simulink model "pendulum"  (Simulink 8.3)
settings: Solver=ode4  StartTime=0.0  StopTime=Tmax  FixedStep=0.01  RelTol=1e-3
values from neighbouring files (symbols this model uses):
  A = [0 0 0 1.0 0 0.16983 0 0 0 0 0 ... (first row only)    [f16_init.m]    (also in pendulum_control_lmi.m = [0         0    1.0000         0; 0         0         0    1; pendulum_init.m = [0 1 0 0; pendulum_init.mat = [0 0 0 0 1 -10.95 0 24.92 0 -2.75 0 28.58 ... (16 elements, ; safety_controller_dynamics.m = [0 1 0 0)
  B = [0 0; 0 0; 0 0; 0 0; 0 0; 0 0; 0 0; 0 0; b71 0; 0 b82; 0 b92]    [f16_init.m]    (also in pendulum_control_lmi.m = [0;0;1.9400;-4.4400]; pendulum_init.m = [0 ; 1.94 ; 0 ; -4.44 ]; pendulum_init.mat = [0 1.94 0 -4.44]; pendulum_nonlinear_init.m = [0; b2; 0; -b4])
  K = K_lmi    [pendulum_init.m]    (also in pendulum_nonlinear_init.m = [7.6, 42.85, 13.54, 8.25]; plot_potential_and_simulation.m = [  0.4072 7.2373  18.6269   3.6725  ]; plot_potential_and_simulation_all_dim.m = [  0.4072 7.2373  18.6269   3.6725  ]; plot_potential_and_simulation_angles.m = [  0.4072 7.2373  18.6269   3.6725  ])
  u_sat_max = va_max    (= 4.95)    [pendulum_init.m]
  u_sat_min = va_min    (= -4.95)    [pendulum_init.m]
  x0 = [ x_init(si); theta_init(si); v_init(si); omega_init(si)]    [pendulum_batch.m]    (also in pendulum_init.m = [-0.170; -0.258; 0.130; 1.170])
  xTerminate = 20    [pendulum_init.m]
  xTerminateMin = 0.02    [pendulum_init.m]
libraries: simulink x2
settings Model: Creator=Fahad  LastModifiedBy=tjohnson
settings DataIOCC: SignalLoggingSaveFormat=Dataset  SignalLogging=off  DSMLogging=off
settings DebuggingCC: AlgebraicLoopMsg=none  SolverPrmCheckMsg=none
settings HardwareCC: ProdIntDivRoundTo=Zero  ProdEndianess=LittleEndian  ProdHWDeviceType=Intel->x86/Pentium
settings RTWCC: GenerateReport=on  RetainRTWFile=on  LaunchReport=on
settings CodeAppCC: ForceParamTrailComments=on  MATLABSourceComments=on
settings GRTTargetCC: CombineOutputUpdateFcns=on  MatFileLogging=off  GRTInterface=off

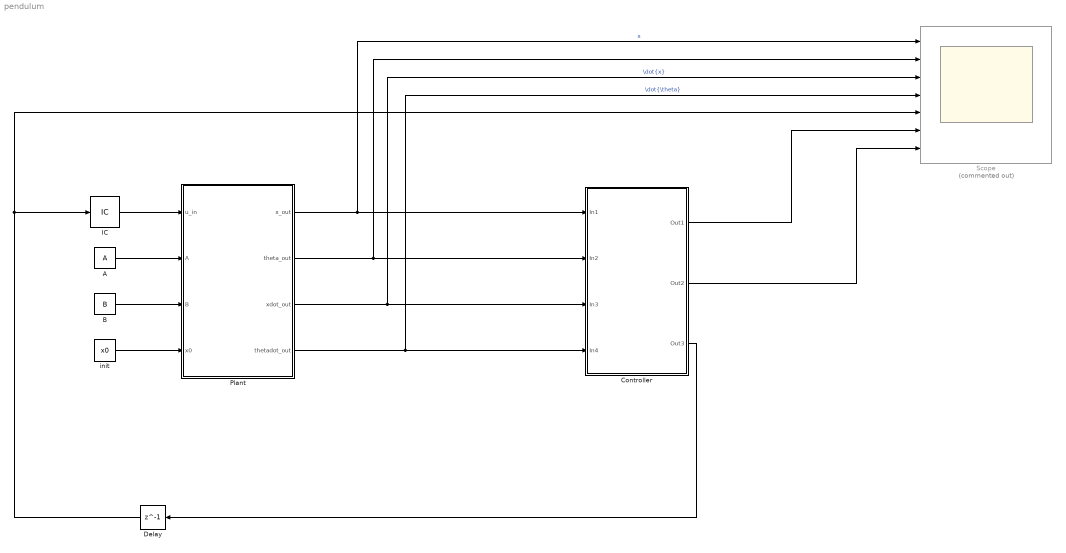
== system pendulum ==
  A : Constant  Value=A
  B : Constant  Value=B
  Controller : Subsystem
  Delay : Delay  DelayLength=1  InitialCondition=0
  IC : InitialCondition  Value=0
  Plant : Stateflow chart  TreatAsAtomicUnit=on
  Scope : Scope  Commented=on  NumInputPorts=7
      settings: ShowLegends=on  TimeRange=15  YMin=-0.07~47.5~0.49~1~4.7025~1.9~-5  YMax=0.02~70~0.6~4~5.1975~2.1~5  SaveName=PendulumScopeData
  init : Constant  Value=x0
  wires:
  Plant/1(x_out) -> Controller/1(In1), Scope/1  "x"
  IC/1 -> Plant/1(u_in)
  Plant/3(xdot_out) -> Scope/3, Controller/3(In3)  "\\dot{x}"
  A/1 -> Plant/2(A)
  B/1 -> Plant/3(B)
  Plant/2(theta_out) -> Scope/2, Controller/2(In2)
  init/1 -> Plant/4(x0)
  Plant/4(thetadot_out) -> Scope/4, Controller/4(In4)  "\\dot{\\theta}"
  Delay/1 -> Scope/5, IC/1
  Controller/1(Out1) -> Scope/6
  Controller/2(Out2) -> Scope/7
  Controller/3(Out3) -> Delay/1

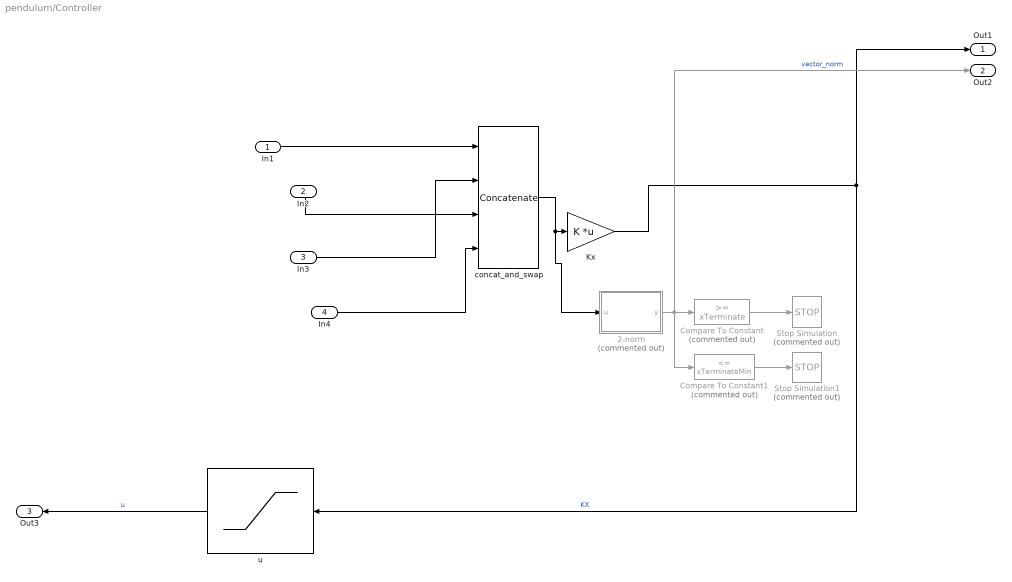
== system pendulum/Controller ==
  In1 : Inport
  In2 : Inport  Port=2
  In3 : Inport  Port=3
  In4 : Inport  Port=4
  2-norm : MATLAB Function  Commented=on  TreatAsAtomicUnit=on
  Compare To Constant : simulink/Logic and Bit Operations/Compare To Constant  Commented=on  relop=>=  const=xTerminate  OutDataTypeStr=boolean
  Compare To Constant1 : simulink/Logic and Bit Operations/Compare To Constant  Commented=on  relop=<=  const=xTerminateMin  OutDataTypeStr=boolean
  Kx : Gain  Gain=K  Multiplication=Matrix(K*u) (u vector)
  Stop Simulation : Stop  Commented=on
  Stop Simulation1 : Stop  Commented=on
  concat_and_swap : Concatenate  NumInputs=4
  u : Saturate  UpperLimit=u_sat_max  LowerLimit=u_sat_min
  Out1 : Outport
  Out2 : Outport  Port=2
  Out3 : Outport  Port=3
  wires:
  Kx/1 -> Out1/1, u/1  "KX"
  u/1 -> Out3/1  "u"
  concat_and_swap/1 -> 2-norm/1(u), Kx/1
  Compare To Constant/1 -> Stop Simulation/1
  2-norm/1(y) -> Out2/1, Compare To Constant1/1, Compare To Constant/1  "vector_norm"
  Compare To Constant1/1 -> Stop Simulation1/1
  In2/1 -> concat_and_swap/3
  In3/1 -> concat_and_swap/2
  In1/1 -> concat_and_swap/1
  In4/1 -> concat_and_swap/4

== stateflow chart Plant ==
  settings: updateMethod=CONTINUOUS
  state Plant
    du:
    x_dot = x*A[0][0]+xdot*A[0][1]+theta*A[0][2]+thetadot*A[0][3]+u_in*B[0];
    xdot_dot = x*A[1][0]+xdot*A[1][1]+theta*A[1][2]+thetadot*A[1][3]+u_in*B[1];
    theta_dot = x*A[2][0]+xdot*A[2][1]+theta*A[2][2]+thetadot*A[2][3]+u_in*B[2];
    thetadot_dot = x*A[3][0]+xdot*A[3][1]+theta*A[3][2]+thetadot*A[3][3]+u_in*B[3];
    x_out = x;
    xdot_out = xdot;
    theta_out = theta;
    thetadot_out = thetadot;
  (default) -> Plant
  data: x local double =x0(1); theta local double =x0(2); xdot local double =x0(3); thetadot local double =x0(4); u_in input double; x_out output double; theta_out output double; xdot_out output double; thetadot_out output double; A input double size=[4 4]; B input double size=[4 1]; x0 input double size=[4 1]
  data x settings: updateMethod=SF_CONTINUOUS_TIME_DATA
  data theta settings: updateMethod=SF_CONTINUOUS_TIME_DATA
  data xdot settings: updateMethod=SF_CONTINUOUS_TIME_DATA
  data thetadot settings: updateMethod=SF_CONTINUOUS_TIME_DATA

== matlab function Controller/2-norm ==
  data: u input double; y output double
function y = fcn(u)
%#codegen

y = norm(u,2);
